simulink model "Q3"  (R2021b)
settings: Solver=VariableStepAuto  StartTime=0.0  StopTime=100  RelTol=1e-3
undefined symbols (not defined in the file): A_numerical, B_numerical, C_numerical, D_numerical, F, K_d_LQR, K_q_LQR, L, L1, Q_1, Q_2, T_O, xd_step
settings Model: Creator=sadeg  LastModifiedBy=sadeg
settings SolverCC: ZeroCrossAlgorithm=Adaptive
settings DebuggingCC: MaskedZcDiagnostic=none  IgnoredZcDiagnostic=none

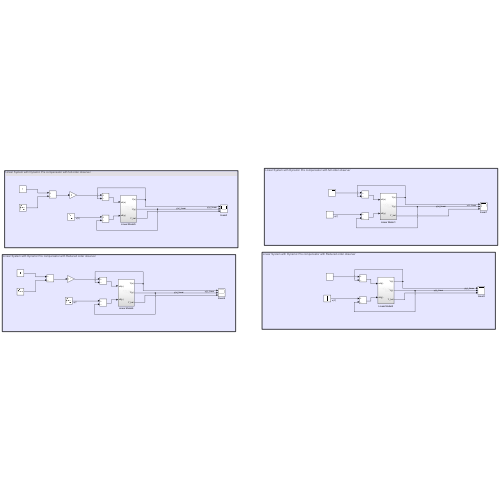
[thumbnail: Simulink's stored preview of the top-level diagram]
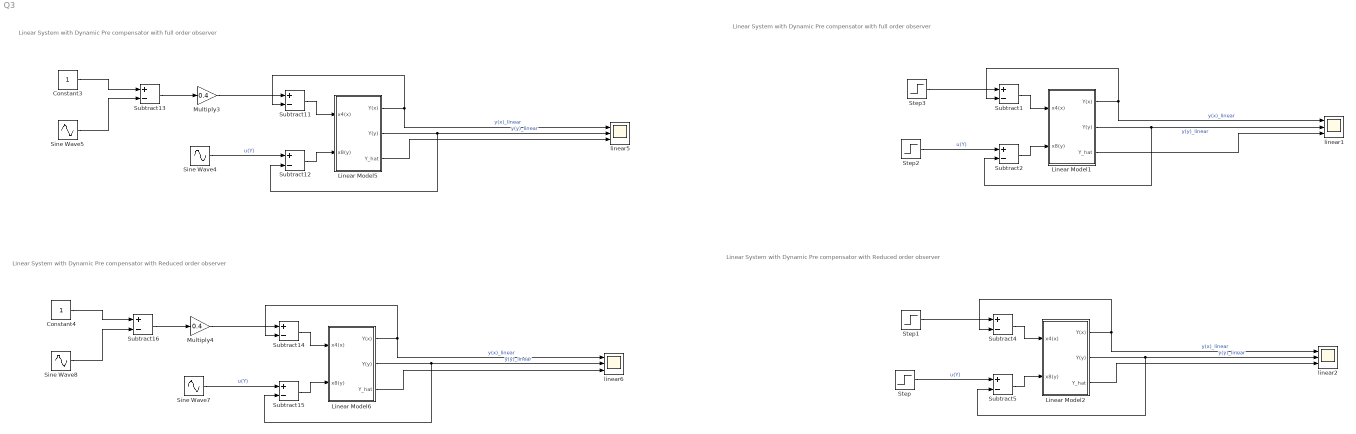
== system Q3 ==
  note: Linear System with Dynamic Pre compensator with full order observer
  note: Linear System with Dynamic Pre compensator with Reduced order observer
  note: Linear System with Dynamic Pre compensator with full order observer
  note: Linear System with Dynamic Pre compensator with Reduced order observer
  Constant3 : Constant
  Constant4 : Constant
  Linear Model1 : Subsystem
  Linear Model2 : Subsystem
  Linear Model5 : Subsystem
  Linear Model6 : Subsystem
  Multiply3 : Gain  Gain=0.4
  Multiply4 : Gain  Gain=0.4
  Sine Wave4 : Sin  Amplitude=0.4  SampleTime=0
  Sine Wave5 : Sin  Phase=pi/2  SampleTime=0
  Sine Wave7 : Sin  Amplitude=0.4  SampleTime=0
  Sine Wave8 : Sin  Phase=pi/2  SampleTime=0
  Step{,1..3} (4 alike) : Step  SampleTime=0
  Subtract{1..2,4..5,11..16} (10 alike) : Sum  Inputs=+-
  linear{1..2,5..6} (4 alike) : Scope  NumInputPorts=3
  wires:
  Subtract13/1 -> Multiply3/1
  Sine Wave5/1 -> Subtract13/2
  Linear Model5/3(Y_hat) -> linear5/3
  Linear Model5/2(Y(y)) -> Subtract12/2, linear5/2  "y(y)_linear"
  Linear Model5/1(Y(x)) -> linear5/1, Subtract11/2  "y(x)_linear"
  Constant3/1 -> Subtract13/1
  Sine Wave4/1 -> Subtract12/1  "u(Y)"
  Subtract11/1 -> Linear Model5/1(x4(x))
  Subtract12/1 -> Linear Model5/2(x8(y))
  Multiply3/1 -> Subtract11/1
  Multiply4/1 -> Subtract14/1
  Subtract15/1 -> Linear Model6/2(x8(y))
  Subtract14/1 -> Linear Model6/1(x4(x))
  Sine Wave7/1 -> Subtract15/1  "u(Y)"
  Constant4/1 -> Subtract16/1
  Linear Model6/3(Y_hat) -> linear6/3
  Linear Model6/1(Y(x)) -> linear6/1, Subtract14/2  "y(x)_linear"
  Sine Wave8/1 -> Subtract16/2
  Linear Model6/2(Y(y)) -> Subtract15/2, linear6/2  "y(y)_linear"
  Subtract16/1 -> Multiply4/1
  Linear Model1/3(Y_hat) -> linear1/3
  Subtract4/1 -> Linear Model2/1(x4(x))
  Linear Model2/2(Y(y)) -> Subtract5/2, linear2/2  "y(y)_linear"
  Linear Model2/1(Y(x)) -> linear2/1, Subtract4/2  "y(x)_linear"
  Subtract5/1 -> Linear Model2/2(x8(y))
  Step/1 -> Subtract5/1  "u(Y)"
  Step2/1 -> Subtract2/1  "u(Y)"
  Subtract1/1 -> Linear Model1/1(x4(x))
  Linear Model2/3(Y_hat) -> linear2/3
  Step3/1 -> Subtract1/1
  Linear Model1/2(Y(y)) -> Subtract2/2, linear1/2  "y(y)_linear"
  Step1/1 -> Subtract4/1
  Subtract2/1 -> Linear Model1/2(x8(y))
  Linear Model1/1(Y(x)) -> Subtract1/2, linear1/1  "y(x)_linear"

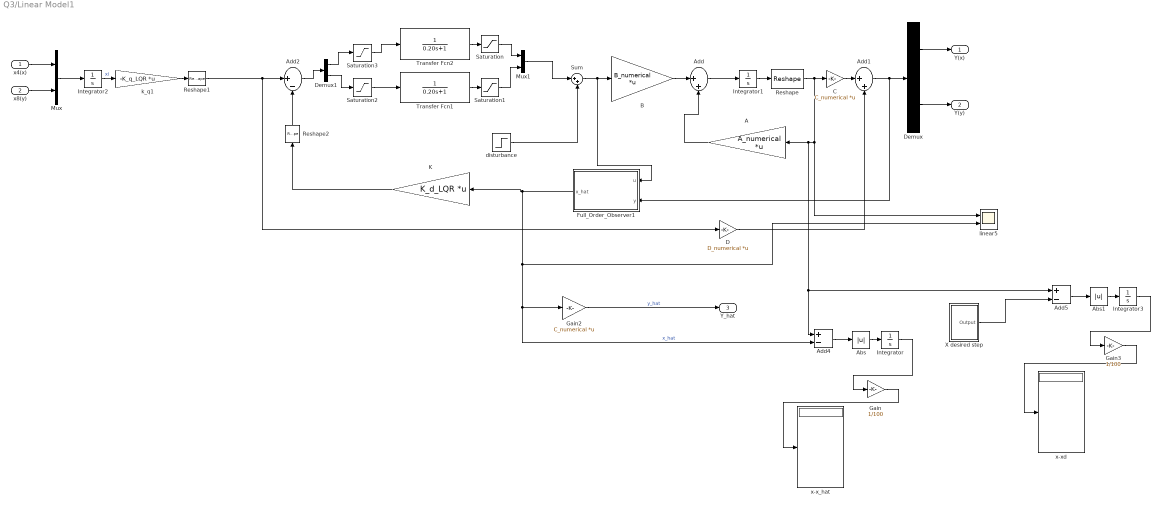
== system Q3/Linear Model1 ==
  x4(x) : Inport
  x8(y) : Inport  Port=2
  A : Gain  Gain=A_numerical  Multiplication=Matrix(K*u)
  Abs : Abs
  Abs1 : Abs
  Add : Sum  Inputs=|++
  Add1 : Sum  Inputs=|++
  Add2 : Sum  Inputs=|+-
  Add4 : Sum  Inputs=+-
  Add5 : Sum  Inputs=+-
  B : Gain  Gain=B_numerical  Multiplication=Matrix(K*u)
  C : Gain  Gain=C_numerical  Multiplication=Matrix(K*u)
  D : Gain  Gain=D_numerical  Multiplication=Matrix(K*u)
  Demux : Demux  Outputs=2
  Demux1 : Demux  Outputs=2
  Full_Order_Observer1 : Subsystem
  Gain : Gain  Gain=1/100
  Gain2 : Gain  Gain=C_numerical  Multiplication=Matrix(K*u)
  Gain3 : Gain  Gain=1/100
  Integrator : Integrator
  Integrator1 : Integrator  InitialCondition=zeros(8,1)
  Integrator2 : Integrator
  Integrator3 : Integrator
  K : Gain  Gain=K_d_LQR  Multiplication=Matrix(K*u)
  Mux : Mux  Inputs=2
  Mux1 : Mux  Inputs=2
  Reshape : Reshape  OutputDimensionality=Column vector (2-D)
  Reshape1 : Reshape  OutputDimensionality=Column vector (2-D)
  Reshape2 : Reshape  OutputDimensionality=Column vector (2-D)
  Saturation : Saturate  UpperLimit=45  LowerLimit=-45
  Saturation1 : Saturate  UpperLimit=45  LowerLimit=-45
  Saturation2 : Saturate  UpperLimit=5  LowerLimit=-5
  Saturation3 : Saturate  UpperLimit=5  LowerLimit=-5
  Sum : Sum  Inputs=|++
  Transfer Fcn1 : TransferFcn  Denominator=[0.20 1]
  Transfer Fcn2 : TransferFcn  Denominator="[0.20  1]"
  X desired step : Subsystem
  disturbance : Step  Time=3  After=0.5  SampleTime=0
  k_q1 : Gain  Gain=-K_q_LQR  Multiplication=Matrix(K*u)
  linear5 : Scope  NumInputPorts=2
  x-x_hat : Display
  x-xd : Display
  Y(x) : Outport
  Y(y) : Outport  Port=2
  Y_hat : Outport  Port=3
  wires:
  Demux/2 -> Y(y)/1
  A/1 -> Add/2
  Integrator1/1 -> Reshape/1
  Reshape/1 -> linear5/1, Add5/1, Add4/1, A/1, C/1
  x4(x)/1 -> Mux/1
  C/1 -> Add1/1
  B/1 -> Add/1
  x8(y)/1 -> Mux/2
  Demux/1 -> Y(x)/1
  Add1/1 -> Full_Order_Observer1/2(y), Demux/1
  Add/1 -> Integrator1/1
  D/1 -> Add1/2
  Reshape1/1 -> D/1, Add2/1
  Mux/1 -> Integrator2/1
  Sum/1 -> Full_Order_Observer1/1(u), B/1
  Integrator2/1 -> k_q1/1  "xi"
  Mux1/1 -> Sum/1
  Add2/1 -> Demux1/1
  Transfer Fcn1/1 -> Saturation1/1
  Saturation1/1 -> Mux1/2
  Transfer Fcn2/1 -> Saturation/1
  Saturation/1 -> Mux1/1
  Saturation2/1 -> Transfer Fcn1/1
  Demux1/2 -> Saturation2/1
  Demux1/1 -> Saturation3/1
  Saturation3/1 -> Transfer Fcn2/1
  disturbance/1 -> Sum/2
  Full_Order_Observer1/1(x_hat) -> linear5/2, Add4/2, Gain2/1, K/1  "x_hat"
  Gain2/1 -> Y_hat/1  "y_hat"
  Add4/1 -> Abs/1
  Abs/1 -> Integrator/1
  Integrator/1 -> Gain/1
  Gain/1 -> x-x_hat/1
  Integrator3/1 -> Gain3/1
  Add5/1 -> Abs1/1
  Gain3/1 -> x-xd/1
  Abs1/1 -> Integrator3/1
  X desired step/1(Output) -> Add5/2
  k_q1/1 -> Reshape1/1
  Reshape2/1 -> Add2/2
  K/1 -> Reshape2/1

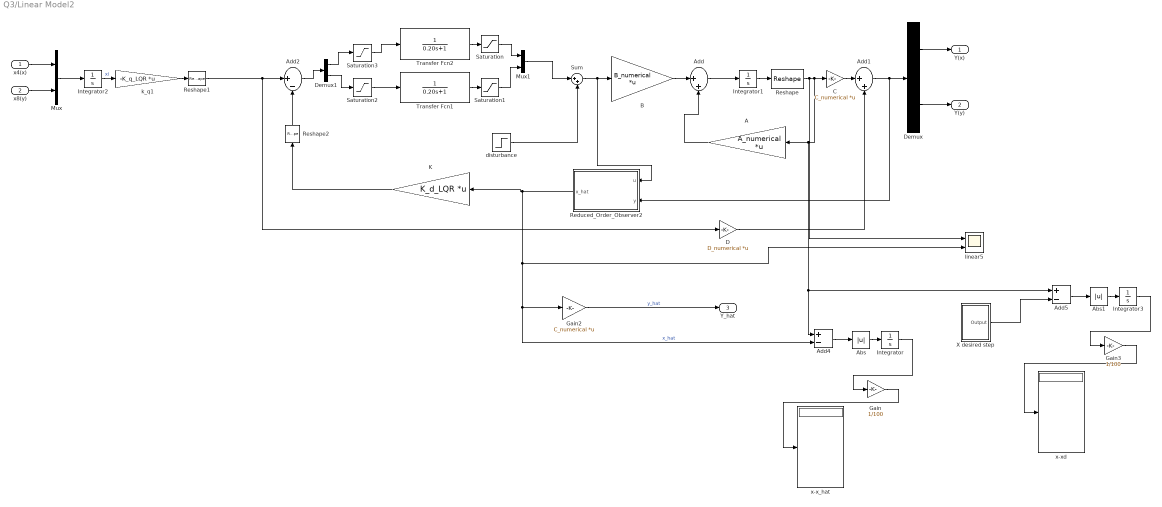
== system Q3/Linear Model2 ==
  x4(x) : Inport
  x8(y) : Inport  Port=2
  A : Gain  Gain=A_numerical  Multiplication=Matrix(K*u)
  Abs : Abs
  Abs1 : Abs
  Add : Sum  Inputs=|++
  Add1 : Sum  Inputs=|++
  Add2 : Sum  Inputs=|+-
  Add4 : Sum  Inputs=+-
  Add5 : Sum  Inputs=+-
  B : Gain  Gain=B_numerical  Multiplication=Matrix(K*u)
  C : Gain  Gain=C_numerical  Multiplication=Matrix(K*u)
  D : Gain  Gain=D_numerical  Multiplication=Matrix(K*u)
  Demux : Demux  Outputs=2
  Demux1 : Demux  Outputs=2
  Gain : Gain  Gain=1/100
  Gain2 : Gain  Gain=C_numerical  Multiplication=Matrix(K*u)
  Gain3 : Gain  Gain=1/100
  Integrator : Integrator
  Integrator1 : Integrator  InitialCondition=zeros(8,1)
  Integrator2 : Integrator
  Integrator3 : Integrator
  K : Gain  Gain=K_d_LQR  Multiplication=Matrix(K*u)
  Mux : Mux  Inputs=2
  Mux1 : Mux  Inputs=2
  Reduced_Order_Observer2 : Subsystem
  Reshape : Reshape  OutputDimensionality=Column vector (2-D)
  Reshape1 : Reshape  OutputDimensionality=Column vector (2-D)
  Reshape2 : Reshape  OutputDimensionality=Column vector (2-D)
  Saturation : Saturate  UpperLimit=45  LowerLimit=-45
  Saturation1 : Saturate  UpperLimit=45  LowerLimit=-45
  Saturation2 : Saturate  UpperLimit=5  LowerLimit=-5
  Saturation3 : Saturate  UpperLimit=5  LowerLimit=-5
  Sum : Sum  Inputs=|++
  Transfer Fcn1 : TransferFcn  Denominator=[0.20 1]
  Transfer Fcn2 : TransferFcn  Denominator="[0.20  1]"
  X desired step : Subsystem
  disturbance : Step  Time=3  After=0.5  SampleTime=0
  k_q1 : Gain  Gain=-K_q_LQR  Multiplication=Matrix(K*u)
  linear5 : Scope  NumInputPorts=2
  x-x_hat : Display
  x-xd : Display
  Y(x) : Outport
  Y(y) : Outport  Port=2
  Y_hat : Outport  Port=3
  wires:
  Demux/2 -> Y(y)/1
  A/1 -> Add/2
  Integrator1/1 -> Reshape/1
  Reshape/1 -> linear5/1, Add5/1, Add4/1, A/1, C/1
  x4(x)/1 -> Mux/1
  C/1 -> Add1/1
  B/1 -> Add/1
  x8(y)/1 -> Mux/2
  Demux/1 -> Y(x)/1
  Add1/1 -> Reduced_Order_Observer2/2(y), Demux/1
  Add/1 -> Integrator1/1
  D/1 -> Add1/2
  Reshape1/1 -> D/1, Add2/1
  Mux/1 -> Integrator2/1
  Sum/1 -> Reduced_Order_Observer2/1(u), B/1
  Integrator2/1 -> k_q1/1  "xi"
  Mux1/1 -> Sum/1
  Add2/1 -> Demux1/1
  Transfer Fcn1/1 -> Saturation1/1
  Saturation1/1 -> Mux1/2
  Transfer Fcn2/1 -> Saturation/1
  Saturation/1 -> Mux1/1
  Saturation2/1 -> Transfer Fcn1/1
  Demux1/2 -> Saturation2/1
  Demux1/1 -> Saturation3/1
  Saturation3/1 -> Transfer Fcn2/1
  disturbance/1 -> Sum/2
  Reduced_Order_Observer2/1(x_hat) -> linear5/2, Add4/2, Gain2/1, K/1  "x_hat"
  Gain2/1 -> Y_hat/1  "y_hat"
  Add4/1 -> Abs/1
  Abs/1 -> Integrator/1
  Integrator/1 -> Gain/1
  Gain/1 -> x-x_hat/1
  Integrator3/1 -> Gain3/1
  Add5/1 -> Abs1/1
  Gain3/1 -> x-xd/1
  Abs1/1 -> Integrator3/1
  X desired step/1(Output) -> Add5/2
  k_q1/1 -> Reshape1/1
  Reshape2/1 -> Add2/2
  K/1 -> Reshape2/1

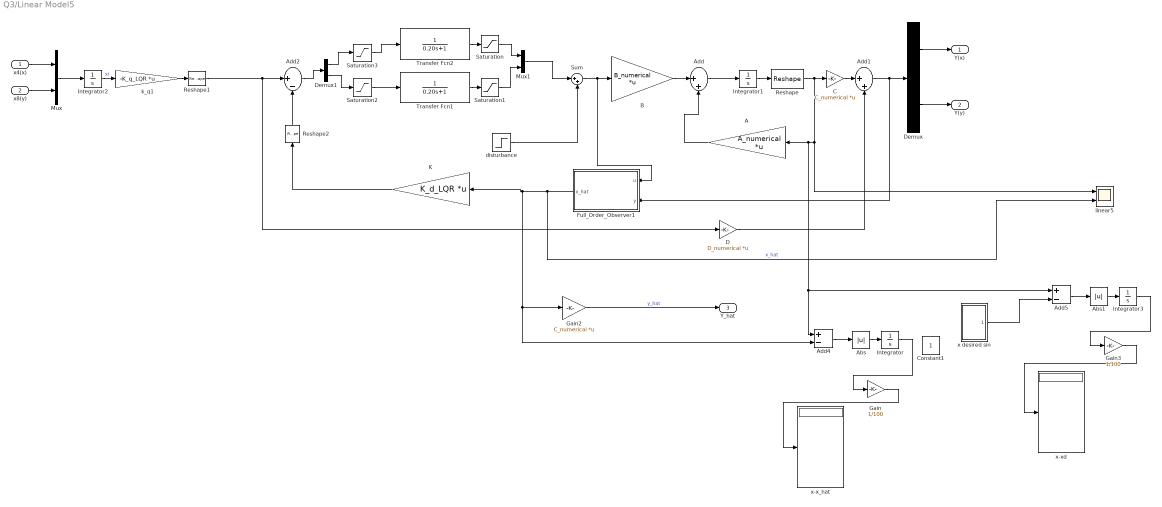
== system Q3/Linear Model5 ==
  x4(x) : Inport
  x8(y) : Inport  Port=2
  A : Gain  Gain=A_numerical  Multiplication=Matrix(K*u)
  Abs : Abs
  Abs1 : Abs
  Add : Sum  Inputs=|++
  Add1 : Sum  Inputs=|++
  Add2 : Sum  Inputs=|+-
  Add4 : Sum  Inputs=+-
  Add5 : Sum  Inputs=+-
  B : Gain  Gain=B_numerical  Multiplication=Matrix(K*u)
  C : Gain  Gain=C_numerical  Multiplication=Matrix(K*u)
  Constant1 : Constant
  D : Gain  Gain=D_numerical  Multiplication=Matrix(K*u)
  Demux : Demux  Outputs=2
  Demux1 : Demux  Outputs=2
  Full_Order_Observer1 : Subsystem
  Gain : Gain  Gain=1/100
  Gain2 : Gain  Gain=C_numerical  Multiplication=Matrix(K*u)
  Gain3 : Gain  Gain=1/100
  Integrator : Integrator
  Integrator1 : Integrator  InitialCondition=zeros(8,1)
  Integrator2 : Integrator
  Integrator3 : Integrator
  K : Gain  Gain=K_d_LQR  Multiplication=Matrix(K*u)
  Mux : Mux  Inputs=2
  Mux1 : Mux  Inputs=2
  Reshape : Reshape  OutputDimensionality=Column vector (2-D)
  Reshape1 : Reshape  OutputDimensionality=Column vector (2-D)
  Reshape2 : Reshape  OutputDimensionality=Column vector (2-D)
  Saturation : Saturate  UpperLimit=45  LowerLimit=-45
  Saturation1 : Saturate  UpperLimit=45  LowerLimit=-45
  Saturation2 : Saturate  UpperLimit=5  LowerLimit=-5
  Saturation3 : Saturate  UpperLimit=5  LowerLimit=-5
  Sum : Sum  Inputs=|++
  Transfer Fcn1 : TransferFcn  Denominator=[0.20 1]
  Transfer Fcn2 : TransferFcn  Denominator="[0.20  1]"
  disturbance : Step  Time=3  After=0.5  SampleTime=0
  k_q1 : Gain  Gain=-K_q_LQR  Multiplication=Matrix(K*u)
  linear5 : Scope  NumInputPorts=2
  x desired sin : Subsystem
  x-x_hat : Display
  x-xd : Display
  Y(x) : Outport
  Y(y) : Outport  Port=2
  Y_hat : Outport  Port=3
  wires:
  Demux/2 -> Y(y)/1
  A/1 -> Add/2
  Integrator1/1 -> Reshape/1
  Reshape/1 -> Add5/1, Add4/1, A/1, linear5/1, C/1
  x4(x)/1 -> Mux/1
  C/1 -> Add1/1
  B/1 -> Add/1
  x8(y)/1 -> Mux/2
  Demux/1 -> Y(x)/1
  Add1/1 -> Full_Order_Observer1/2(y), Demux/1
  Add/1 -> Integrator1/1
  D/1 -> Add1/2
  Reshape1/1 -> D/1, Add2/1
  Mux/1 -> Integrator2/1
  Sum/1 -> Full_Order_Observer1/1(u), B/1
  Integrator2/1 -> k_q1/1  "xi"
  Mux1/1 -> Sum/1
  Add2/1 -> Demux1/1
  Transfer Fcn1/1 -> Saturation1/1
  Saturation1/1 -> Mux1/2
  Transfer Fcn2/1 -> Saturation/1
  Saturation/1 -> Mux1/1
  Saturation2/1 -> Transfer Fcn1/1
  Demux1/2 -> Saturation2/1
  Demux1/1 -> Saturation3/1
  Saturation3/1 -> Transfer Fcn2/1
  disturbance/1 -> Sum/2
  Full_Order_Observer1/1(x_hat) -> linear5/2, Add4/2, Gain2/1, K/1  "x_hat"
  Gain2/1 -> Y_hat/1  "y_hat"
  Add4/1 -> Abs/1
  Abs/1 -> Integrator/1
  Integrator/1 -> Gain/1
  Gain/1 -> x-x_hat/1
  Integrator3/1 -> Gain3/1
  Add5/1 -> Abs1/1
  Gain3/1 -> x-xd/1
  Abs1/1 -> Integrator3/1
  x desired sin/1(Output) -> Add5/2
  k_q1/1 -> Reshape1/1
  Reshape2/1 -> Add2/2
  K/1 -> Reshape2/1

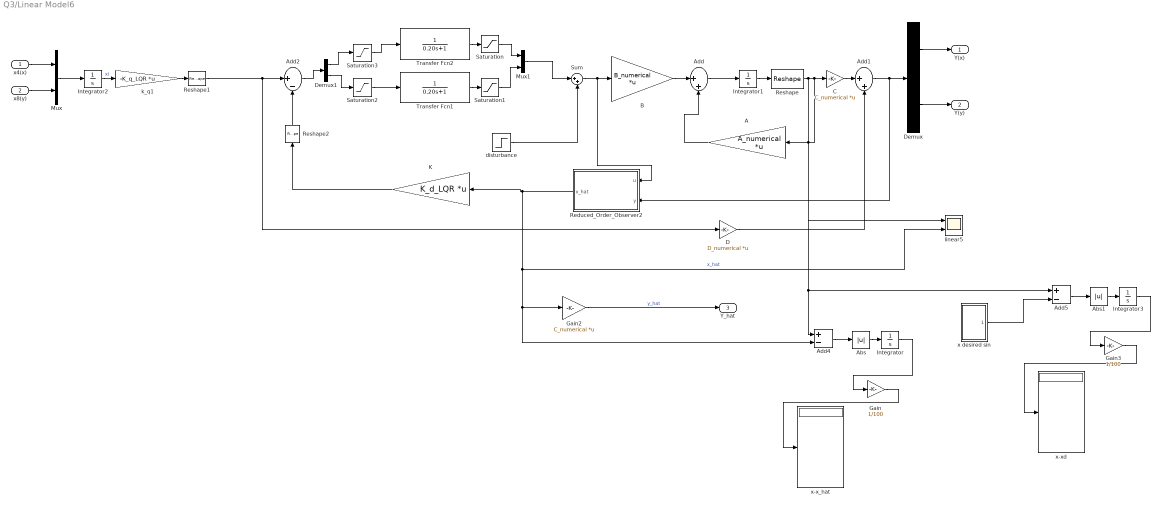
== system Q3/Linear Model6 ==
  x4(x) : Inport
  x8(y) : Inport  Port=2
  A : Gain  Gain=A_numerical  Multiplication=Matrix(K*u)
  Abs : Abs
  Abs1 : Abs
  Add : Sum  Inputs=|++
  Add1 : Sum  Inputs=|++
  Add2 : Sum  Inputs=|+-
  Add4 : Sum  Inputs=+-
  Add5 : Sum  Inputs=+-
  B : Gain  Gain=B_numerical  Multiplication=Matrix(K*u)
  C : Gain  Gain=C_numerical  Multiplication=Matrix(K*u)
  D : Gain  Gain=D_numerical  Multiplication=Matrix(K*u)
  Demux : Demux  Outputs=2
  Demux1 : Demux  Outputs=2
  Gain : Gain  Gain=1/100
  Gain2 : Gain  Gain=C_numerical  Multiplication=Matrix(K*u)
  Gain3 : Gain  Gain=1/100
  Integrator : Integrator
  Integrator1 : Integrator  InitialCondition=zeros(8,1)
  Integrator2 : Integrator
  Integrator3 : Integrator
  K : Gain  Gain=K_d_LQR  Multiplication=Matrix(K*u)
  Mux : Mux  Inputs=2
  Mux1 : Mux  Inputs=2
  Reduced_Order_Observer2 : Subsystem
  Reshape : Reshape  OutputDimensionality=Column vector (2-D)
  Reshape1 : Reshape  OutputDimensionality=Column vector (2-D)
  Reshape2 : Reshape  OutputDimensionality=Column vector (2-D)
  Saturation : Saturate  UpperLimit=45  LowerLimit=-45
  Saturation1 : Saturate  UpperLimit=45  LowerLimit=-45
  Saturation2 : Saturate  UpperLimit=5  LowerLimit=-5
  Saturation3 : Saturate  UpperLimit=5  LowerLimit=-5
  Sum : Sum  Inputs=|++
  Transfer Fcn1 : TransferFcn  Denominator=[0.20 1]
  Transfer Fcn2 : TransferFcn  Denominator="[0.20  1]"
  disturbance : Step  Time=3  After=0.5  SampleTime=0
  k_q1 : Gain  Gain=-K_q_LQR  Multiplication=Matrix(K*u)
  linear5 : Scope  NumInputPorts=2
  x desired sin : Subsystem
  x-x_hat : Display
  x-xd : Display
  Y(x) : Outport
  Y(y) : Outport  Port=2
  Y_hat : Outport  Port=3
  wires:
  Demux/2 -> Y(y)/1
  A/1 -> Add/2
  Integrator1/1 -> Reshape/1
  Reshape/1 -> linear5/1, Add5/1, Add4/1, A/1, C/1
  x4(x)/1 -> Mux/1
  C/1 -> Add1/1
  B/1 -> Add/1
  x8(y)/1 -> Mux/2
  Demux/1 -> Y(x)/1
  Add1/1 -> Reduced_Order_Observer2/2(y), Demux/1
  Add/1 -> Integrator1/1
  D/1 -> Add1/2
  Reshape1/1 -> D/1, Add2/1
  Mux/1 -> Integrator2/1
  Sum/1 -> Reduced_Order_Observer2/1(u), B/1
  Integrator2/1 -> k_q1/1  "xi"
  Mux1/1 -> Sum/1
  Add2/1 -> Demux1/1
  Transfer Fcn1/1 -> Saturation1/1
  Saturation1/1 -> Mux1/2
  Transfer Fcn2/1 -> Saturation/1
  Saturation/1 -> Mux1/1
  Saturation2/1 -> Transfer Fcn1/1
  Demux1/2 -> Saturation2/1
  Demux1/1 -> Saturation3/1
  Saturation3/1 -> Transfer Fcn2/1
  disturbance/1 -> Sum/2
  Reduced_Order_Observer2/1(x_hat) -> linear5/2, Add4/2, Gain2/1, K/1  "x_hat"
  Gain2/1 -> Y_hat/1  "y_hat"
  Add4/1 -> Abs/1
  Abs/1 -> Integrator/1
  Integrator/1 -> Gain/1
  Gain/1 -> x-x_hat/1
  Integrator3/1 -> Gain3/1
  Add5/1 -> Abs1/1
  Gain3/1 -> x-xd/1
  Abs1/1 -> Integrator3/1
  x desired sin/1(Output) -> Add5/2
  k_q1/1 -> Reshape1/1
  Reshape2/1 -> Add2/2
  K/1 -> Reshape2/1

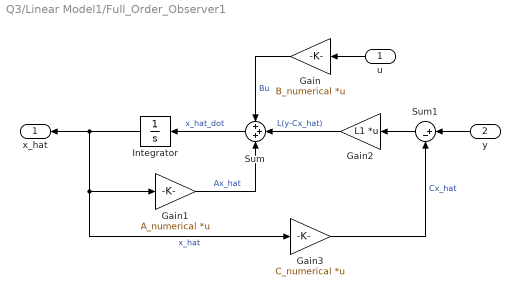
== system Q3/Linear Model1/Full_Order_Observer1 ==
  u : Inport
  y : Inport  Port=2
  Gain : Gain  Gain=B_numerical  Multiplication=Matrix(K*u)
  Gain1 : Gain  Gain=A_numerical  Multiplication=Matrix(K*u)
  Gain2 : Gain  Gain=L1  Multiplication=Matrix(K*u)
  Gain3 : Gain  Gain=C_numerical  Multiplication=Matrix(K*u)
  Integrator : Integrator
  Sum : Sum  Inputs=+++
  Sum1 : Sum  Inputs=|+-
  x_hat : Outport
  wires:
  u/1 -> Gain/1
  Sum/1 -> Integrator/1  "x_hat_dot"
  Gain/1 -> Sum/1  "Bu"
  Integrator/1 -> x_hat/1, Gain3/1, Gain1/1  "x_hat"
  Gain1/1 -> Sum/3  "Ax_hat"
  y/1 -> Sum1/1
  Gain2/1 -> Sum/2  "L(y-Cx_hat)"
  Sum1/1 -> Gain2/1
  Gain3/1 -> Sum1/2  "Cx_hat"

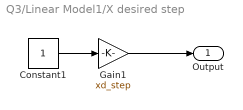
== system Q3/Linear Model1/X desired step ==
  Constant1 : Constant
  Gain1 : Gain  Gain=xd_step
  Output : Outport
  wires:
  Constant1/1 -> Gain1/1
  Gain1/1 -> Output/1

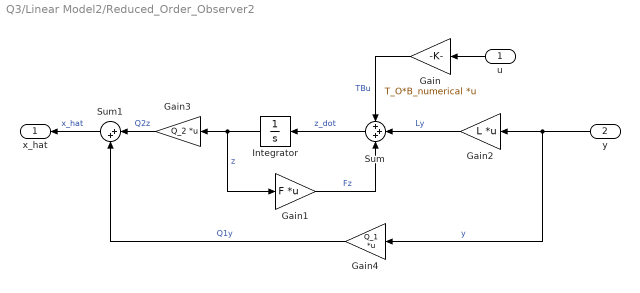
== system Q3/Linear Model2/Reduced_Order_Observer2 ==
  u : Inport
  y : Inport  Port=2
  Gain : Gain  Gain=T_O*B_numerical  Multiplication=Matrix(K*u)
  Gain1 : Gain  Gain=F  Multiplication=Matrix(K*u)
  Gain2 : Gain  Gain=L  Multiplication=Matrix(K*u)
  Gain3 : Gain  Gain=Q_2  Multiplication=Matrix(K*u)
  Gain4 : Gain  Gain=Q_1  Multiplication=Matrix(K*u)
  Integrator : Integrator
  Sum : Sum  Inputs=+++
  Sum1 : Sum  Inputs=|++
  x_hat : Outport
  wires:
  u/1 -> Gain/1
  Sum/1 -> Integrator/1  "z_dot"
  Gain/1 -> Sum/1  "TBu"
  Integrator/1 -> Gain3/1, Gain1/1  "z"
  Gain1/1 -> Sum/3  "Fz"
  Gain2/1 -> Sum/2  "Ly"
  y/1 -> Gain4/1, Gain2/1  "y"
  Sum1/1 -> x_hat/1  "x_hat"
  Gain3/1 -> Sum1/1  "Q2z"
  Gain4/1 -> Sum1/2  "Q1y"

== system Q3/Linear Model2/X desired step ==
  Constant1 : Constant
  Gain1 : Gain  Gain=xd_step
  Output : Outport
  wires:
  Constant1/1 -> Gain1/1
  Gain1/1 -> Output/1

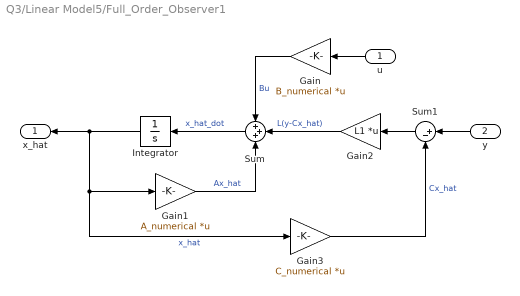
== system Q3/Linear Model5/Full_Order_Observer1 ==
  u : Inport
  y : Inport  Port=2
  Gain : Gain  Gain=B_numerical  Multiplication=Matrix(K*u)
  Gain1 : Gain  Gain=A_numerical  Multiplication=Matrix(K*u)
  Gain2 : Gain  Gain=L1  Multiplication=Matrix(K*u)
  Gain3 : Gain  Gain=C_numerical  Multiplication=Matrix(K*u)
  Integrator : Integrator
  Sum : Sum  Inputs=+++
  Sum1 : Sum  Inputs=|+-
  x_hat : Outport
  wires:
  u/1 -> Gain/1
  Sum/1 -> Integrator/1  "x_hat_dot"
  Gain/1 -> Sum/1  "Bu"
  Integrator/1 -> x_hat/1, Gain3/1, Gain1/1  "x_hat"
  Gain1/1 -> Sum/3  "Ax_hat"
  y/1 -> Sum1/1
  Gain2/1 -> Sum/2  "L(y-Cx_hat)"
  Sum1/1 -> Gain2/1
  Gain3/1 -> Sum1/2  "Cx_hat"

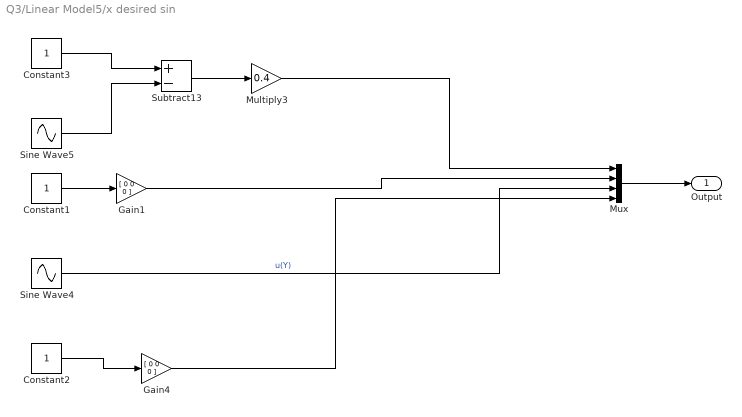
== system Q3/Linear Model5/x desired sin ==
  Constant1 : Constant
  Constant2 : Constant
  Constant3 : Constant
  Gain1 : Gain  Gain=[ 0 0 0 ]
  Gain4 : Gain  Gain=[ 0 0 0 ]
  Multiply3 : Gain  Gain=0.4
  Mux : Mux
  Sine Wave4 : Sin  Amplitude=0.4  SampleTime=0
  Sine Wave5 : Sin  Phase=pi/2  SampleTime=0
  Subtract13 : Sum  Inputs=+-
  Output : Outport
  wires:
  Constant3/1 -> Subtract13/1
  Multiply3/1 -> Mux/1
  Constant1/1 -> Gain1/1
  Constant2/1 -> Gain4/1
  Sine Wave4/1 -> Mux/3  "u(Y)"
  Subtract13/1 -> Multiply3/1
  Gain4/1 -> Mux/4
  Sine Wave5/1 -> Subtract13/2
  Gain1/1 -> Mux/2
  Mux/1 -> Output/1

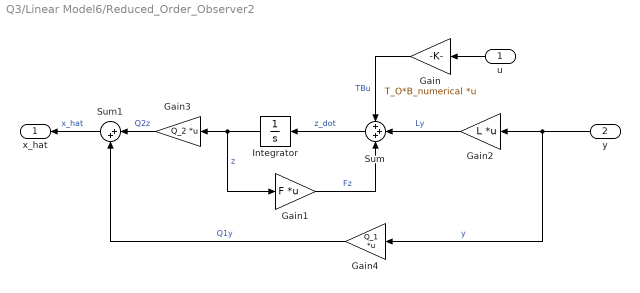
== system Q3/Linear Model6/Reduced_Order_Observer2 ==
  u : Inport
  y : Inport  Port=2
  Gain : Gain  Gain=T_O*B_numerical  Multiplication=Matrix(K*u)
  Gain1 : Gain  Gain=F  Multiplication=Matrix(K*u)
  Gain2 : Gain  Gain=L  Multiplication=Matrix(K*u)
  Gain3 : Gain  Gain=Q_2  Multiplication=Matrix(K*u)
  Gain4 : Gain  Gain=Q_1  Multiplication=Matrix(K*u)
  Integrator : Integrator
  Sum : Sum  Inputs=+++
  Sum1 : Sum  Inputs=|++
  x_hat : Outport
  wires:
  u/1 -> Gain/1
  Sum/1 -> Integrator/1  "z_dot"
  Gain/1 -> Sum/1  "TBu"
  Integrator/1 -> Gain3/1, Gain1/1  "z"
  Gain1/1 -> Sum/3  "Fz"
  Gain2/1 -> Sum/2  "Ly"
  y/1 -> Gain4/1, Gain2/1  "y"
  Sum1/1 -> x_hat/1  "x_hat"
  Gain3/1 -> Sum1/1  "Q2z"
  Gain4/1 -> Sum1/2  "Q1y"

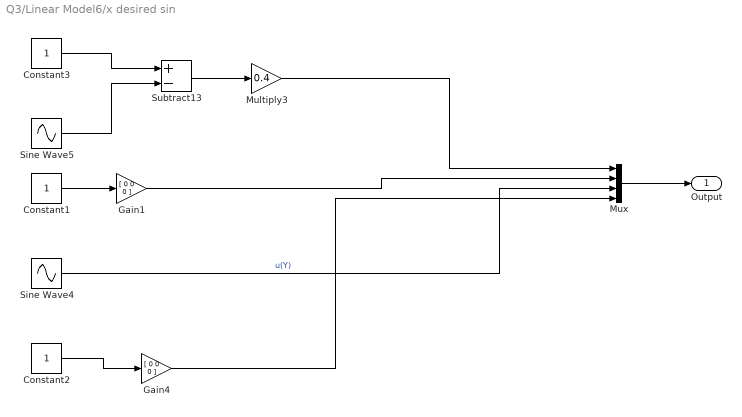
== system Q3/Linear Model6/x desired sin ==
  Constant1 : Constant
  Constant2 : Constant
  Constant3 : Constant
  Gain1 : Gain  Gain=[ 0 0 0 ]
  Gain4 : Gain  Gain=[ 0 0 0 ]
  Multiply3 : Gain  Gain=0.4
  Mux : Mux
  Sine Wave4 : Sin  Amplitude=0.4  SampleTime=0
  Sine Wave5 : Sin  Phase=pi/2  SampleTime=0
  Subtract13 : Sum  Inputs=+-
  Output : Outport
  wires:
  Constant3/1 -> Subtract13/1
  Multiply3/1 -> Mux/1
  Constant1/1 -> Gain1/1
  Constant2/1 -> Gain4/1
  Sine Wave4/1 -> Mux/3  "u(Y)"
  Subtract13/1 -> Multiply3/1
  Gain4/1 -> Mux/4
  Sine Wave5/1 -> Subtract13/2
  Gain1/1 -> Mux/2
  Mux/1 -> Output/1
